simulink model "Dynamic_Leg_Model_1"  (R2018b)
settings: Solver=ode45  StartTime=0.0  StopTime=100.0  MaxStep=0.1  RelTol=1e-3
settings Model: Creator=jabyrns2  LastModifiedBy=jabyrns2
settings DebuggingCC: UnderSpecifiedDimensionMsg=warning

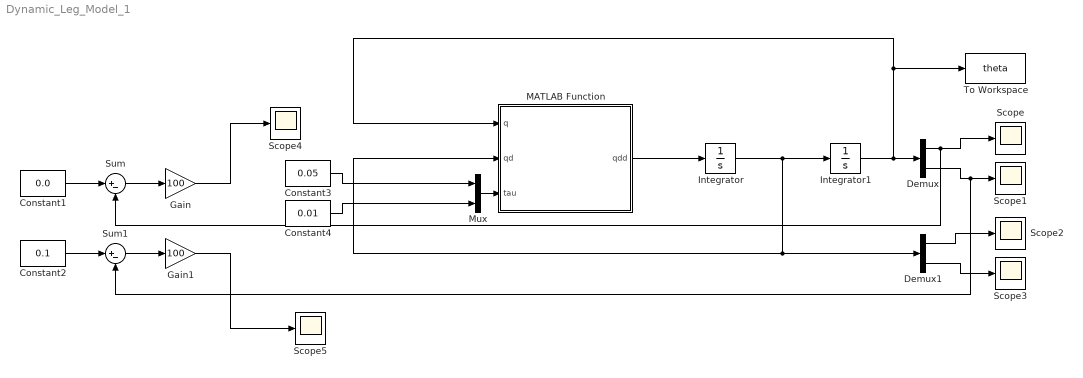
== system Dynamic_Leg_Model_1 ==
  Constant1 : Constant  Value=0.0
  Constant2 : Constant  Value=0.1
  Constant3 : Constant  Value=0.05
  Constant4 : Constant  Value=0.01
  Demux : Demux  Outputs=2
  Demux1 : Demux  Outputs=2
  Gain : Gain  Gain=100
  Gain1 : Gain  Gain=100
  Integrator : Integrator  InitialCondition=[0;0]
  Integrator1 : Integrator  InitialCondition=[0;0]
  MATLAB Function : MATLAB Function  TreatAsAtomicUnit=on
  Mux : Mux  Inputs=2
  Scope{,1..5} (6 alike) : Scope
  Sum : Sum  Inputs=|+-
  Sum1 : Sum  Inputs=|+-
  To Workspace : ToWorkspace  VariableName=theta  SampleTime=-1
  wires:
  Integrator/1 -> Demux1/1, MATLAB Function/2(qd), Integrator1/1
  Integrator1/1 -> To Workspace/1, MATLAB Function/1(q), Demux/1
  Demux/1 -> Scope/1, Sum/2
  Demux/2 -> Scope1/1, Sum1/2
  Demux1/1 -> Scope2/1
  Demux1/2 -> Scope3/1
  Mux/1 -> MATLAB Function/3(tau)
  Gain/1 -> Scope4/1
  Gain1/1 -> Scope5/1
  MATLAB Function/1(qdd) -> Integrator/1
  Constant1/1 -> Sum/1
  Sum/1 -> Gain/1
  Constant2/1 -> Sum1/1
  Sum1/1 -> Gain1/1
  Constant4/1 -> Mux/2
  Constant3/1 -> Mux/1

== matlab function Dynamic_Leg_Model_1/MATLAB Function ==
  data: q input; qdd output; qd input; tau input
function qdd = fcn(q, qd, tau)
    t1 = q(1);
    t2 = q(2);
    t1d = qd(1);
    t2d = qd(2);
    tau1 = tau(1);
    tau2 = tau(2);

    l1 = 0.215; % 215mm
    l2 = 0.215; % 215mm
    lc1 = 0.05; % 50mm ---CHANGE
    lc2 = 0.10; % 100mm  ---CHANGE
    m1 = 0.950; % 950 grams ---CHANGE
    m2 = 0.100; % 100 grams ---CHANGE
    i1 = 0.01;
    i2 = 0.5;

    p1 = m1*lc1 + m2*lc1*lc1 + i1;
    p2 = m2*lc2*lc2 + i2;
    p3 = m2*l1*lc2;
    p4 = m1*lc1*m2*l1;
    p5 = m2*lc2;

    D = [p1 + p2 + 2*p3*cos(t2) , p2 + p3*cos(t2); p2 + p3*cos(t2) , p2];

    C = [-p3*sin(t2)*t2d , -p3*sin(t2)*t2d - p3*sin(t2)*t1d; p3*sin(t2)*t1d , 0];

    G = [-p4*(-9.81)*cos(t1) - p5*(-9.81)*cos(t1 + t2) ; -p5*(-9.81)*cos(t1 + t2)];
    
    qdd = inv(D)*[tau1;tau2]-inv(D)*C*qd - inv(D)*G;
end
